simulink model "ue_1_a"  (R2015b)
settings: Solver=VariableStepAuto  StartTime=0.0  StopTime=10.0  RelTol=1e-3
settings Model: Creator=dbarelop  LastModifiedBy=dbarelop

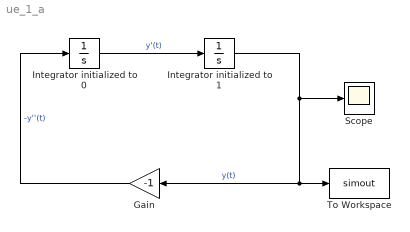
== system ue_1_a ==
  Gain : Gain  Gain=-1
  Integrator initialized to 0 : Integrator
  Integrator initialized to 1 : Integrator  InitialCondition=1
  Scope : Scope
  To Workspace : ToWorkspace  VariableName=simout  SaveFormat=Timeseries  SampleTime=-1
  wires:
  Integrator initialized to 0/1 -> Integrator initialized to 1/1  "y'(t)"
  Integrator initialized to 1/1 -> Scope/1, Gain/1, To Workspace/1  "y(t)"
  Gain/1 -> Integrator initialized to 0/1  "-y''(t)"
